simulink model "sampleModel2006"  (R2023a)
settings: Solver=VariableStepAuto  StartTime=0.0  StopTime=10.0  RelTol=1e-3
libraries: hdlsllib x8
settings Model: Creator=user1  LastModifiedBy=user1

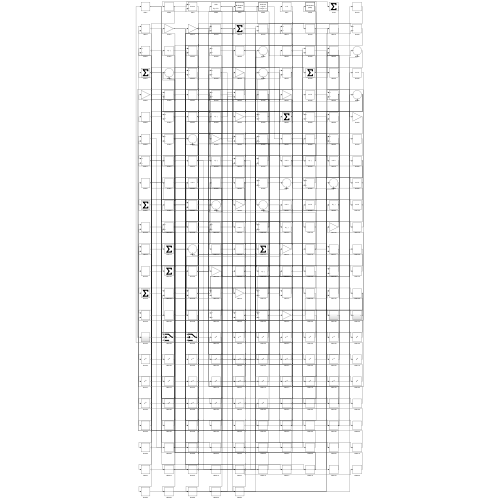
[thumbnail: Simulink's stored preview of the top-level diagram]
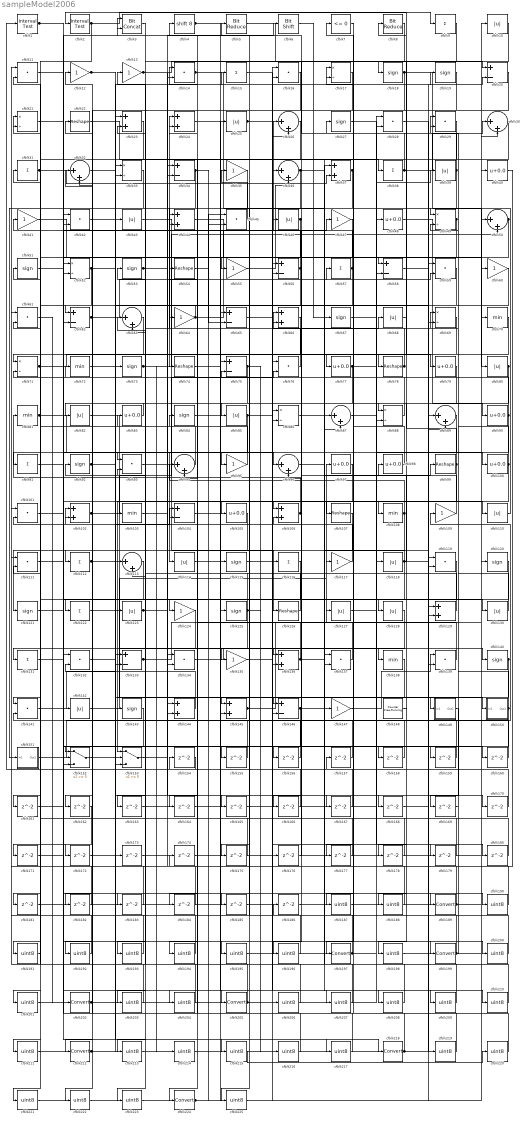
== system sampleModel2006 ==
  cfblk1 : hdlsllib/Logic and Bit Operations/Interval Test  IntervalClosedRight=on  uplimit=0.5  IntervalClosedLeft=on  lowlimit=-0.5  OutDataTypeStr=boolean
  cfblk{10,25,39,43,46,68,80,82,85,110,114,118,123,127..128,130,142} (17 alike) : Abs  SaturateOnIntegerOverflow=off
  cfblk{40,48,77,79,83,90,97..98,100,105} (10 alike) : Bias  Bias=0.0  SaturateOnIntegerOverflow=off
  cfblk{11,14,16,28..29,42,45,59,61,76,93,101,111,119,132,134,137,139,141} (19 alike) : DotProduct  OutDataTypeStr=Inherit: Inherit via internal rule
  cfblk{23..24,37,44,66,102,106,129,136,144..145} (11 alike) : Sum
  cfblk{70,72,81,103,108,138} (6 alike) : MinMax
  cfblk{20,34,56,58,62,65,75,104,133,146} (10 alike) : Sum  Inputs=+-
  cfblk{22,54,74,78,99,107,126} (7 alike) : Reshape
  cfblk{12..13,35,41,47,55,60,64,95,109,117,124,135,147} (14 alike) : Gain
  cfblk{9,15,31,38,57,91,112,116,122,131} (10 alike) : Sum  Inputs=+
  cfblk{26,30,32,36,50,63,87,89,94,96,113} (11 alike) : Sum  Inputs=|++
  cfblk{18..19,27,51,53,67,73,84,92,115,120..121,125,140,143} (15 alike) : Signum
  cfblk148 : hdlsllib/Sources/Counter Free-Running  NumBits=16  tsamp=-1
  cfblk149 : Subsystem
      settings: LibrarySourceBlock=|
      | hdlsllib/Ports &
      | Subsystems/Subsystem
  cfblk150 : Subsystem
      settings: LibrarySourceBlock=|
      | hdlsllib/Ports &
      | Subsystems/Subsystem
  cfblk151 : Subsystem
      settings: LibrarySourceBlock=|
      | hdlsllib/Ports &
      | Subsystems/Subsystem
  cfblk152 : Switch  SaturateOnIntegerOverflow=off  InputSameDT=off
  cfblk153 : Switch  SaturateOnIntegerOverflow=off  InputSameDT=off
  cfblk{154..186} (33 alike) : Delay  SampleTime=1
  cfblk{17,21,33,49,52,69,71,86,88} (9 alike) : Product  Inputs=*/  RndMeth=Zero  SaturateOnIntegerOverflow=on
  cfblk{187..188,190..196,198,200..201,203..204,206..211,213..217,219..223,225} (31 alike) : DataTypeConversion  OutDataTypeStr=uint8  SaturateOnIntegerOverflow=off  RndMeth=Floor
  cfblk{189,197,199,202,205,212,218,224} (8 alike) : DataTypeConversion  SaturateOnIntegerOverflow=off  RndMeth=Floor
  cfblk2 : hdlsllib/Logic and Bit Operations/Interval Test  IntervalClosedRight=on  uplimit=0.5  IntervalClosedLeft=on  lowlimit=-0.5  OutDataTypeStr=boolean
  cfblk3 : hdlsllib/Logic and Bit Operations/Bit Concat  numInputs=2
  cfblk4 : ArithShift  BitShiftNumber=8
  cfblk5 : hdlsllib/Logic and Bit Operations/Bit Reduce  mode=AND
  cfblk6 : hdlsllib/Logic and Bit Operations/Bit Shift  mode=Shift Left Logical  N=0
  cfblk7 : hdlsllib/Logic and Bit Operations/Compare To Zero  relop=<=  OutDataTypeStr=boolean
  cfblk8 : hdlsllib/Logic and Bit Operations/Bit Reduce  mode=AND
  wires:
  cfblk82/1 -> cfblk150/1(In1)
  cfblk105/1 -> cfblk121/1
  cfblk34/1 -> cfblk151/1(In1), cfblk65/2
  cfblk151/1(Out1) -> cfblk109/1
  cfblk120/1 -> cfblk224/1
  cfblk90/1 -> cfblk114/1, cfblk21/1
  cfblk6/1 -> cfblk67/1
  cfblk54/1 -> cfblk45/1
  cfblk125/1 -> cfblk83/1, cfblk134/2, cfblk176/1
  cfblk62/1 -> cfblk57/1, cfblk17/1
  cfblk68/1 -> cfblk2/1
  cfblk73/1 -> cfblk50/2, cfblk214/1
  cfblk24/1 -> cfblk147/1
  cfblk95/1 -> cfblk51/1
  cfblk71/1 -> cfblk77/1, cfblk128/1
  cfblk1/1 -> cfblk108/1, cfblk56/2
  cfblk56/1 -> cfblk41/1, cfblk143/1
  cfblk110/1 -> cfblk49/1
  cfblk18/1 -> cfblk60/1, cfblk86/2
  cfblk64/1 -> cfblk26/1, cfblk62/1
  cfblk129/1 -> cfblk92/1
  cfblk48/1 -> cfblk90/1
  cfblk38/1 -> cfblk30/1, cfblk3/1
  cfblk140/1 -> cfblk177/1, cfblk178/1
  cfblk43/1 -> cfblk126/1
  cfblk126/1 -> cfblk63/1
  cfblk137/1 -> cfblk97/1
  cfblk14/1 -> cfblk38/1, cfblk79/1
  cfblk145/1 -> cfblk40/1, cfblk175/1
  cfblk88/1 -> cfblk27/1
  cfblk81/1 -> cfblk93/1, cfblk3/2
  cfblk41/1 -> cfblk55/1
  cfblk80/1 -> cfblk88/1, cfblk105/1
  cfblk19/1 -> cfblk146/1
  cfblk2/1 -> cfblk9/1, cfblk161/1
  cfblk134/1 -> cfblk140/1
  cfblk49/1 -> cfblk129/2, cfblk94/2
  cfblk100/1 -> cfblk153/1, cfblk66/2
  cfblk12/1 -> cfblk149/1(In1), cfblk168/1
  cfblk93/1 -> cfblk75/2
  cfblk33/1 -> cfblk52/2
  cfblk30/1 -> cfblk78/1
  cfblk74/1 -> cfblk116/1
  cfblk4/1 -> cfblk130/1, cfblk158/1
  cfblk44/1 -> cfblk80/1
  cfblk117/1 -> cfblk31/1
  cfblk96/1 -> cfblk119/2
  cfblk106/1 -> cfblk81/1, cfblk66/1
  cfblk97/1 -> cfblk124/1
  cfblk85/1 -> cfblk131/1, cfblk68/1, cfblk123/1
  cfblk70/1 -> cfblk197/1
  cfblk76/1 -> cfblk24/1
  cfblk26/1 -> cfblk71/1
  cfblk51/1 -> cfblk47/1
  cfblk36/1 -> cfblk74/1, cfblk87/2
  cfblk135/1 -> cfblk36/1
  cfblk127/1 -> cfblk28/2
  cfblk122/1 -> cfblk137/2
  cfblk147/1 -> cfblk139/1
  cfblk9/1 -> cfblk58/1
  cfblk104/1 -> cfblk25/1
  cfblk22/1 -> cfblk87/1
  cfblk118/1 -> cfblk141/1, cfblk112/1, cfblk98/1, cfblk20/2
  cfblk77/1 -> cfblk39/1, cfblk122/1
  cfblk20/1 -> cfblk33/2
  cfblk101/1 -> cfblk189/1
  cfblk116/1 -> cfblk153/2
  cfblk52/1 -> cfblk91/1, cfblk69/2
  cfblk102/1 -> cfblk76/2, cfblk19/1
  cfblk31/1 -> cfblk37/2, cfblk95/1
  cfblk146/1 -> cfblk152/3, cfblk209/1
  cfblk42/1 -> cfblk199/1
  cfblk15/1 -> cfblk146/2
  cfblk8/1 -> cfblk103/1
  cfblk144/1 -> cfblk102/1
  cfblk141/1 -> cfblk73/1
  cfblk45/1 -> cfblk35/1
  cfblk92/1 -> cfblk15/1, cfblk107/1
  cfblk99/1 -> cfblk8/1, cfblk166/1
  cfblk10/1 -> cfblk106/1
  cfblk98/1 -> cfblk44/1
  cfblk61/1 -> cfblk202/1
  cfblk114/1 -> cfblk65/1
  cfblk83/1 -> cfblk82/1
  cfblk111/1 -> cfblk142/1
  cfblk108/1 -> cfblk94/1, cfblk225/1
  cfblk11/1 -> cfblk205/1
  cfblk55/1 -> cfblk36/2
  cfblk39/1 -> cfblk85/1, cfblk17/2
  cfblk152/1 -> cfblk113/1
  cfblk29/1 -> cfblk64/1
  cfblk53/1 -> cfblk59/2, cfblk193/1
  cfblk69/1 -> cfblk136/1
  cfblk87/1 -> cfblk100/1
  cfblk13/1 -> cfblk20/1, cfblk145/2
  cfblk25/1 -> cfblk138/1, cfblk167/1
  cfblk109/1 -> cfblk46/1
  cfblk150/1(Out1) -> cfblk69/1, cfblk145/1, cfblk164/1
  cfblk46/1 -> cfblk162/1, cfblk213/1
  cfblk3/1 -> cfblk113/2
  cfblk16/1 -> cfblk212/1
  cfblk17/1 -> cfblk153/3
  cfblk142/1 -> cfblk117/1
  cfblk132/1 -> cfblk218/1
  cfblk78/1 -> cfblk44/2, cfblk53/1
  cfblk37/1 -> cfblk133/2, cfblk156/1
  cfblk35/1 -> cfblk144/2
  cfblk91/1 -> cfblk96/1
  cfblk123/1 -> cfblk34/2, cfblk135/1, cfblk6/1
  cfblk139/1 -> cfblk14/1
  cfblk5/1 -> cfblk18/1
  cfblk112/1 -> cfblk104/1, cfblk204/1
  cfblk133/1 -> cfblk10/1, cfblk58/2
  cfblk130/1 -> cfblk29/1
  cfblk50/1 -> cfblk152/2, cfblk62/2, cfblk201/1
  cfblk94/1 -> cfblk22/1
  cfblk75/1 -> cfblk216/1, cfblk223/1
  cfblk27/1 -> cfblk110/1
  cfblk57/1 -> cfblk152/1, cfblk21/2
  cfblk136/1 -> cfblk99/1, cfblk104/2
  cfblk154/1 -> cfblk1/1
  cfblk60/1 -> cfblk155/1
  cfblk155/1 -> cfblk141/2
  cfblk156/1 -> cfblk24/2
  cfblk157/1 -> cfblk102/2
  cfblk158/1 -> cfblk76/1
  cfblk131/1 -> cfblk159/1
  cfblk159/1 -> cfblk129/1
  cfblk58/1 -> cfblk160/1
  cfblk160/1 -> cfblk93/2
  cfblk59/1 -> cfblk163/1
  cfblk163/1 -> cfblk88/2
  cfblk164/1 -> cfblk86/1
  cfblk103/1 -> cfblk165/1
  cfblk165/1 -> cfblk136/2
  cfblk166/1 -> cfblk111/2
  cfblk167/1 -> cfblk34/1
  cfblk168/1 -> cfblk119/1
  cfblk149/1(Out1) -> cfblk169/1
  cfblk169/1 -> cfblk49/2
  cfblk153/1 -> cfblk170/1
  cfblk170/1 -> cfblk37/1
  cfblk66/1 -> cfblk171/1
  cfblk143/1 -> cfblk172/1
  cfblk172/1 -> cfblk50/1
  cfblk173/1 -> cfblk14/2
  cfblk40/1 -> cfblk174/1
  cfblk174/1 -> cfblk26/2
  cfblk175/1 -> cfblk133/1
  cfblk176/1 -> cfblk106/2
  cfblk177/1 -> cfblk75/1
  cfblk178/1 -> cfblk63/2
  cfblk65/1 -> cfblk179/1
  cfblk179/1 -> cfblk96/2
  cfblk67/1 -> cfblk180/1
  cfblk180/1 -> cfblk71/2
  cfblk124/1 -> cfblk181/1
  cfblk181/1 -> cfblk30/2
  cfblk128/1 -> cfblk182/1
  cfblk182/1 -> cfblk52/1
  cfblk21/1 -> cfblk183/1
  cfblk183/1 -> cfblk33/1
  cfblk107/1 -> cfblk184/1
  cfblk184/1 -> cfblk144/1
  cfblk121/1 -> cfblk185/1
  cfblk186/1 -> cfblk139/2
  cfblk7/1 -> cfblk187/1
  cfblk187/1 -> cfblk48/1
  cfblk148/1 -> cfblk188/1
  cfblk188/1 -> cfblk7/1
  cfblk189/1 -> cfblk134/1, cfblk54/1
  cfblk86/1 -> cfblk190/1
  cfblk190/1 -> cfblk101/1
  cfblk162/1 -> cfblk191/1
  cfblk191/1 -> cfblk101/2
  cfblk23/1 -> cfblk192/1
  cfblk192/1 -> cfblk111/1
  cfblk193/1 -> cfblk23/1
  cfblk119/1 -> cfblk194/1
  cfblk194/1 -> cfblk23/2
  cfblk72/1 -> cfblk195/1
  cfblk195/1 -> cfblk28/1
  cfblk47/1 -> cfblk196/1
  cfblk196/1 -> cfblk72/1
  cfblk197/1 -> cfblk186/1, cfblk127/1
  cfblk79/1 -> cfblk198/1
  cfblk198/1 -> cfblk70/1
  cfblk199/1 -> cfblk29/2, cfblk5/1
  cfblk171/1 -> cfblk200/1
  cfblk200/1 -> cfblk42/1
  cfblk201/1 -> cfblk42/2
  cfblk202/1 -> cfblk173/1, cfblk56/1, cfblk12/1
  cfblk138/1 -> cfblk203/1
  cfblk203/1 -> cfblk61/1
  cfblk204/1 -> cfblk61/2
  cfblk205/1 -> cfblk154/1, cfblk118/1
  cfblk206/1 -> cfblk11/1
  cfblk185/1 -> cfblk207/1
  cfblk207/1 -> cfblk11/2
  cfblk84/1 -> cfblk208/1
  cfblk208/1 -> cfblk13/1
  cfblk209/1 -> cfblk84/1
  cfblk115/1 -> cfblk210/1
  cfblk210/1 -> cfblk137/1
  cfblk113/1 -> cfblk211/1
  cfblk211/1 -> cfblk115/1
  cfblk212/1 -> cfblk43/1, cfblk59/1
  cfblk213/1 -> cfblk16/1
  cfblk214/1 -> cfblk16/2
  cfblk32/1 -> cfblk215/1
  cfblk216/1 -> cfblk32/1
  cfblk161/1 -> cfblk217/1
  cfblk217/1 -> cfblk32/2
  cfblk218/1 -> cfblk157/1, cfblk4/1
  cfblk28/1 -> cfblk219/1
  cfblk219/1 -> cfblk132/1
  cfblk215/1 -> cfblk220/1
  cfblk220/1 -> cfblk132/2
  cfblk89/1 -> cfblk221/1
  cfblk221/1 -> cfblk125/1
  cfblk63/1 -> cfblk222/1
  cfblk222/1 -> cfblk89/1
  cfblk223/1 -> cfblk89/2
  cfblk224/1 -> cfblk206/1, cfblk45/2
  cfblk225/1 -> cfblk120/1

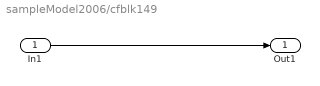
== system sampleModel2006/cfblk149 ==
  In1 : Inport
  Out1 : Outport
  wires:
  In1/1 -> Out1/1

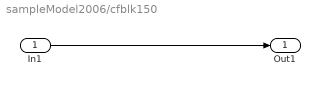
== system sampleModel2006/cfblk150 ==
  In1 : Inport
  Out1 : Outport
  wires:
  In1/1 -> Out1/1

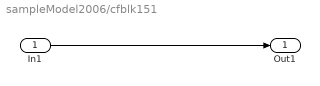
== system sampleModel2006/cfblk151 ==
  In1 : Inport
  Out1 : Outport
  wires:
  In1/1 -> Out1/1
